simulink model "PF_implementacion_PI_Flujo"  (R2023a)
settings: Solver=ode15s  StartTime=0.0  StopTime=t_sim  RelTol=1e-3
values from neighbouring files (symbols this model uses):
  F_in = 2.9843    [PF_CP_Completo_PID.m]    (also in PF_Sfunction2_L.m = u(1); PF_Sfunction2_NL.m = u(1))
  I0_in_fin = I0_in    (= 200)    [PF_CP_Completo_PID.m]
  I0_in_ini = I0_in    (= 200)    [PF_CP_Completo_PID.m]
  L_in_fin = L_in    (= 0)    [PF_CP_Completo_PID.m]
  L_in_ini = L_in    (= 0)    [PF_CP_Completo_PID.m]
  L_ss = ODE_ss(5)    [PF_CP_Completo_PID.m]
  L_ss_ini = L_ss*0.5    [PF_CP_Completo_PID.m]
  Q_in_fin = Q_in    (= 0)    [PF_CP_Completo_PID.m]
  Q_in_ini = Q_in    (= 0)    [PF_CP_Completo_PID.m]
  S1_in_fin = S1_in*1.5    (= 90)    [PF_CP_Completo_PID.m]
  S1_in_ini = S1_in    (= 60)    [PF_CP_Completo_PID.m]
  S2_in_fin = S2_in    (= 20)    [PF_CP_Completo_PID.m]
  S2_in_ini = S2_in    (= 20)    [PF_CP_Completo_PID.m]
  t_sp_change = 5000    [PF_CP_Completo_PID.m]
  t_step = 2000    [PF_CP_Completo_PID.m]
  x_in_fin = x_in    (= 0)    [PF_CP_Completo_PID.m]
  x_in_ini = x_in    (= 0)    [PF_CP_Completo_PID.m]
libraries: slpidlib x1
settings Model: Creator=ja616  LastModifiedBy=ja616

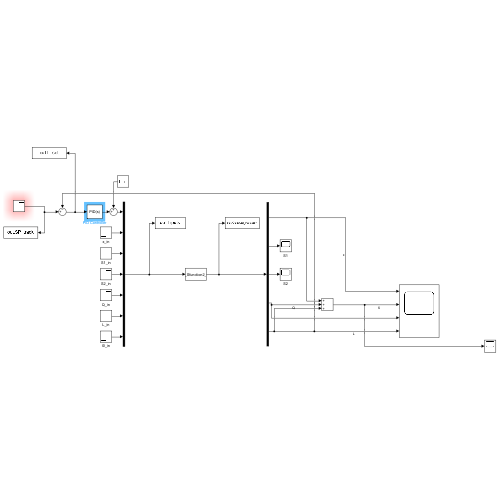
[thumbnail: Simulink's stored preview of the top-level diagram]
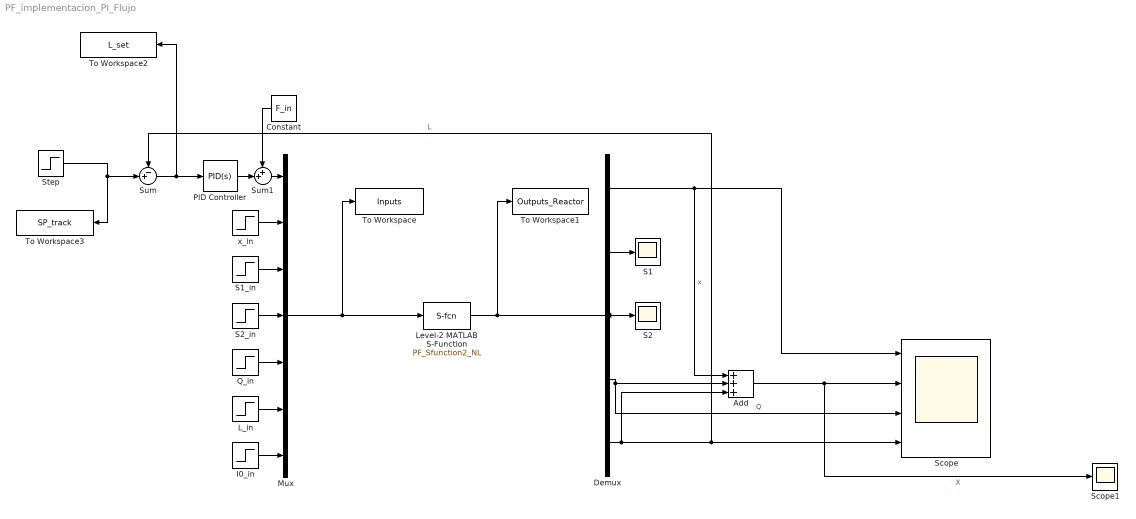
== system PF_implementacion_PI_Flujo ==
  Add : Sum  Inputs=+++
  Constant : Constant  Value=F_in
  Demux : Demux  Outputs=5
  I0_in : Step  Time=t_step  Before=I0_in_ini  After=I0_in_fin  SampleTime=0
  L_in : Step  Time=t_step  Before=L_in_ini  After=L_in_fin  SampleTime=0
  Level-2 MATLAB S-Function : M-S-Function  FunctionName=PF_Sfunction2_NL
  Mux : Mux  Inputs=7
  PID Controller : slpidlib/PID Controller  Controller=PID  Form=Parallel  TimeDomain=Continuous-time  UseExternalTs=off  SampleTime=-1  IntegratorMethod=Forward Euler  FilterMethod=Forward Euler  ControllerParametersSource=internal  P=1.97417255687863  I=0.00156153648825557  UseKiTs=off  D=-263.005534671874  N=0.00750620156850162  UseFilter=on  TunerSelectOption=Transfer Function Based (PID Tuner App)  InitialConditionSource=internal  InitialConditionForIntegrator=0  InitialConditionForFilter=0  DifferentiatorICPrevScaledInput=0  ExternalReset=none  TrackingMode=off  Kt=1  LimitOutput=off  SatLimitsSource=internal  UpperSaturationLimit=inf  LowerSaturationLimit=-inf  LinearizeAsGain=on  AntiWindupMode=none  Kb=1  LimitIntegrator=off  UpperIntegratorSaturationLimit=inf  LowerIntegratorSaturationLimit=-inf  POutMin=[]  POutMax=[]  IOutMin=[]  IOutMax=[]  DOutMin=[]  DOutMax=[]  NOutMin=[]  NOutMax=[]  SumOutMin=[]  SumOutMax=[]  SaturationOutMin=[]  SaturationOutMax=[]  PParamMin=[]  PParamMax=[]  IParamMin=[]  IParamMax=[]  DParamMin=[]  DParamMax=[]  NParamMin=[]  NParamMax=[]  KbParamMin=[]  KbParamMax=[]  KtParamMin=[]  KtParamMax=[]  KbOutMin=[]  KbOutMax=[]  KtOutMin=[]  KtOutMax=[]  IntegratorOutMin=[]  IntegratorOutMax=[]  FilterOutMin=[]  FilterOutMax=[]  SumI1OutMin=[]  SumI1OutMax=[]  SumI2OutMin=[]  SumI2OutMax=[]  SumI3OutMin=[]  SumI3OutMax=[]  SumI4OutMin=[]  SumI4OutMax=[]  SumDOutMin=[]  SumDOutMax=[]  DifferentiatorOutMin=[]  DifferentiatorOutMax=[]  FilterDiffOutCoefMin=[]  FilterDiffOutCoefMax=[]  ReciprocalOutMin=[]  ReciprocalOutMax=[]  SumDenOutMin=[]  SumDenOutMax=[]  SumNumOutMin=[]  SumNumOutMax=[]  DivideOutMin=[]  DivideOutMax=[]  UdiffTsProdOutMin=[]  UdiffTsProdOutMax=[]  NTsProdOutMin=[]  NTsProdOutMax=[]  UintegralTsProdOutMin=[]  UintegralTsProdOutMax=[]  UngainTsProdOutMin=[]  UngainTsProdOutMax=[]  ClampingZeroOutDataTypeStr=Inherit: Inherit via back propagation  ClampingZeroOutMin=[]  ClampingZeroOutMax=[]  FilterDenConstantOutDataTypeStr=Inherit: Inherit via back propagation  FilterDenConstantOutMin=[]  FilterDenConstantOutMax=[]  PCopyOutDataTypeStr=Inherit: Inherit via back propagation  PCopyOutMin=[]  PCopyOutMax=[]  NCopyOutDataTypeStr=Inherit: Inherit via back propagation  NCopyOutMin=[]  NCopyOutMax=[]  IntegratorContinuousStateAttributes=''  IntegratorStateMustResolveToSignalObject=off  IntegratorRTWStateStorageClass=Auto  FilterContinuousStateAttributes=''  FilterStateMustResolveToSignalObject=off  FilterRTWStateStorageClass=Auto  ParallelPVariant=InternalParameters  IdealPVariant=Disabled  IVariant=InternalParameters  DVariant=InternalParameters  IntegratorVariant=Continuous  SatVariant=Disabled  AWVariant=Passthrough  PCopyVariant=Disabled  TRVariant=Disabled  FdbkBlocksVariant=Forward  IdealPFdbkVariant=Disabled  SatFdbkVariant=Disabled  DerivativeFilterVariant=ContFilter  NVariant=InternalParameters  NCopyVariant=Disabled  FilterICVariant=InternalICsFilter  IntegratorICVariant=InternalICs  ExternalResetVariant=Disabled  TRSumVariant=Passthrough  SumFdbkVariant=Disabled  SumVariant=Sum_PID  TsampFilterVariant=InternalTs  TsampNgainVariant=Passthrough  TsampIntegralVariant=Disabled_SignalSpec  ExternalSaturationOutDataTypeStr=Inherit: Same as second input
  Q_in : Step  Time=t_step  Before=Q_in_ini  After=Q_in_fin  SampleTime=0
  S1 : Scope
  S1_in : Step  Time=t_step  Before=S1_in_ini  After=S1_in_fin  SampleTime=0
  S2 : Scope
  S2_in : Step  Time=t_step  Before=S2_in_ini  After=S2_in_fin  SampleTime=0
  Scope : Scope  NumInputPorts=4
  Scope1 : Scope
  Step : Step  Time=t_sp_change  Before=L_ss_ini  After=L_ss  SampleTime=0
  Sum : Sum  Inputs=-+|
  Sum1 : Sum  Inputs=++|
  To Workspace : ToWorkspace  VariableName=Inputs  SaveFormat=Timeseries  SampleTime=-1
  To Workspace1 : ToWorkspace  VariableName=Outputs_Reactor  SaveFormat=Timeseries  SampleTime=-1
  To Workspace2 : ToWorkspace  VariableName=L_set  SaveFormat=Timeseries  SampleTime=-1
  To Workspace3 : ToWorkspace  VariableName=SP_track  SaveFormat=Timeseries  SampleTime=-1
  x_in : Step  Time=t_step  Before=x_in_ini  After=x_in_fin  SampleTime=0
  wires:
  Mux/1 -> Level-2 MATLAB S-Function/1, To Workspace/1
  L_in/1 -> Mux/6
  S2_in/1 -> Mux/4
  Level-2 MATLAB S-Function/1 -> Demux/1, To Workspace1/1
  Q_in/1 -> Mux/5
  x_in/1 -> Mux/2
  Demux/1 -> Scope/1, Add/1  "x"
  Demux/2 -> S1/1
  Demux/3 -> S2/1
  Demux/4 -> Scope/3, Add/2  "Q"
  Demux/5 -> Add/3, Scope/4, Sum/1  "L"
  Add/1 -> Scope1/1, Scope/2  "X"
  I0_in/1 -> Mux/7
  Sum/1 -> To Workspace2/1, PID Controller/1
  Step/1 -> To Workspace3/1, Sum/2
  S1_in/1 -> Mux/3
  PID Controller/1 -> Sum1/2
  Sum1/1 -> Mux/1
  Constant/1 -> Sum1/1
